simulink model "Calculator Simulink"  (R2016a)
settings: Solver=FixedStepDiscrete  StartTime=0.0  StopTime=10.0  RelTol=1e-3
settings Model: Creator=pc  LastModifiedBy=pc
settings OptimizationCC: DefaultParameterBehavior=Inlined  OptimizeModelRefInitCode=on  LifeSpan=1
settings RTWCC: SystemTargetFile=ert.tlc  GenCodeOnly=on  GenerateMakefile=off  TemplateMakefile=ert_default_tmf  GenerateReport=on  IncludeHyperlinkInReport=on  LaunchReport=on  GenerateTraceInfo=on  GenerateTraceReport=on  GenerateTraceReportSl=on  GenerateTraceReportSf=on  GenerateTraceReportEml=on
settings CodeAppCC: ForceParamTrailComments=on  IgnoreCustomStorageClasses=off  OperatorAnnotations=on  SimulinkDataObjDesc=on  SFDataObjDesc=on  MATLABFcnDesc=on  InsertBlockDesc=on  MATLABSourceComments=on
settings ERTTargetCC: GenerateSampleERTMain=on  SuppressErrorStatus=on  InlinedParameterPlacement=NonHierarchical  ERTCustomFileTemplate=example_file_process.tlc  EnableUserReplacementTypes=on

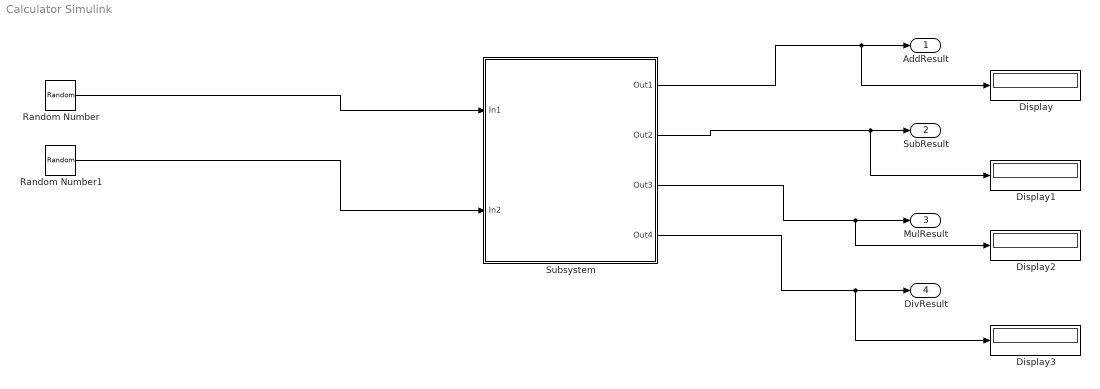
== system Calculator Simulink ==
  Display{,1..3} (4 alike) : Display
  Random Number : RandomNumber  Variance=5  SampleTime=0.1
  Random Number1 : RandomNumber  SampleTime=0.1
  Subsystem : Subsystem
  AddResult : Outport
  SubResult : Outport  Port=2
  MulResult : Outport  Port=3
  DivResult : Outport  Port=4
  wires:
  Random Number/1 -> Subsystem/1(In1)
  Random Number1/1 -> Subsystem/2(In2)
  Subsystem/1(Out1) -> Display/1, AddResult/1
  Subsystem/2(Out2) -> Display1/1, SubResult/1
  Subsystem/3(Out3) -> Display2/1, MulResult/1
  Subsystem/4(Out4) -> Display3/1, DivResult/1

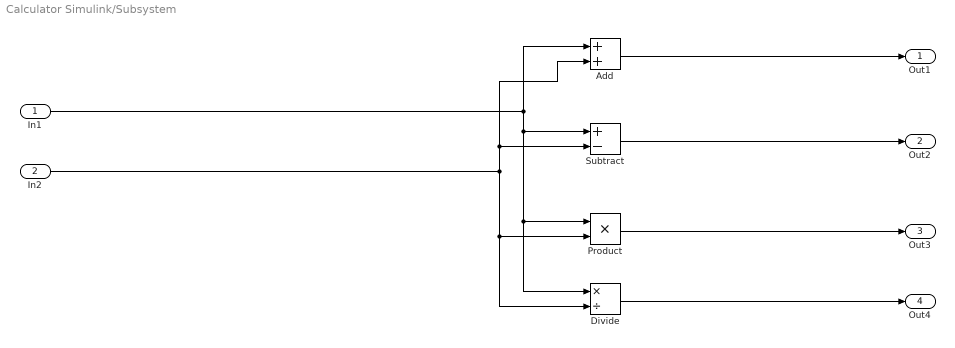
== system Calculator Simulink/Subsystem ==
  In1 : Inport
  In2 : Inport  Port=2
  Add : Sum
  Divide : Product  Inputs=*/
  Product : Product
  Subtract : Sum  Inputs=+-
  Out1 : Outport
  Out2 : Outport  Port=2
  Out3 : Outport  Port=3
  Out4 : Outport  Port=4
  wires:
  Add/1 -> Out1/1
  Product/1 -> Out3/1
  Divide/1 -> Out4/1
  Subtract/1 -> Out2/1
  In2/1 -> Add/2, Subtract/2, Divide/2, Product/2
  In1/1 -> Add/1, Divide/1, Product/1, Subtract/1
